simulink model "test_matlab_system_19"  (Simulink 10.0)
settings: Solver=FixedStepAuto  StartTime=0.0  StopTime=Config.simulationTime  FixedStep=Config.tStep  RelTol=1e-3
PostLoadFcn:
  | % Set path to the utility functions and to WBC library
  | import wbc.*
  | addpath(genpath('./src'));
  | addpath('./lib/RobotDynamicsWithContacts');
InitFcn:
  | init
undefined symbols (not defined in the file or in its folder): Config, confVisualizer
libraries: robotDynamicsWithContacts_lib x1
settings Model: Creator=giuseppe  LastModifiedBy=nunoguedelha
settings DataIOCC: SaveFormat=Dataset  ReturnWorkspaceOutputs=on
settings OptimizationCC: LifeSpan=auto
settings DebuggingCC: UnderspecifiedInitializationDetection=Simplified  MergeDetectMultiDrivingBlocksExec=error  SFUnexpectedBacktrackingDiag=error  SFNoUnconditionalDefaultTransitionDiag=error  SFExecutionAtInitializationDiag=warning  ArithmeticOperatorsInVariantConditions=error
settings HardwareCC: ProdBitPerPointer=64  ProdBitPerSizeT=64  ProdBitPerPtrDiffT=64  ProdLargestAtomicFloat=Float  ProdIntDivRoundTo=Zero  ProdEndianess=LittleEndian  ProdWordSize=64  ProdHWDeviceType=Intel->x86-64 (Windows64)
settings ModelReferenceCC: PropagateSignalLabelsOutOfModel=on
settings SFSimCC: SimUseLocalCustomCode=on  CustomCodeUndefinedFunction=FilterOut
settings RTWCC: RTWUseLocalCustomCode=on
settings CodeAppCC: StateflowObjectComments=off
settings GRTTargetCC: TargetLangStandard=C99 (ISO)  CombineOutputUpdateFcns=on  GRTInterface=off
settings ConfigComp: CovMetricSettings=dwe  CovHtmlReporting=off  CovSaveCumulativeToWorkspaceVar=off  CovSaveSingleToWorkspaceVar=off

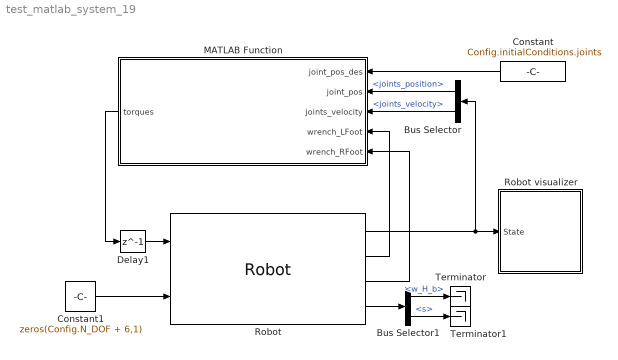
== system test_matlab_system_19 ==
  Bus Selector : BusSelector  OutputSignals=joints_position,joints_velocity
  Bus Selector1 : BusSelector  OutputSignals=w_H_b,s
  Constant : Constant  Value=Config.initialConditions.joints
  Constant1 : Constant  Value=zeros(Config.N_DOF + 6,1)
  Delay1 : Delay  DelayLength=1  InitialCondition=zeros(23,1)
  MATLAB Function : MATLAB Function  TreatAsAtomicUnit=on
  Robot : robotDynamicsWithContacts_lib/Robot  SystemSampleTime=-1  Latency=0  AutoFrameSizeCalculation=off
      settings: SourceProductName=RobotDynamicsWithContacts
  Robot visualizer : Subsystem  SystemSampleTime=confVisualizer.tStep
  Terminator : Terminator
  Terminator1 : Terminator
  wires:
  Constant1/1 -> Robot/2
  Bus Selector/1 -> MATLAB Function/2(joint_pos)  "<joints_position>"
  Bus Selector/2 -> MATLAB Function/3(joints_velocity)  "<joints_velocity>"
  Robot/1 -> Robot visualizer/1(State), Bus Selector/1
  Robot/2 -> MATLAB Function/4(wrench_LFoot)
  Robot/3 -> MATLAB Function/5(wrench_RFoot)
  Constant/1 -> MATLAB Function/1(joint_pos_des)
  MATLAB Function/1(torques) -> Delay1/1
  Delay1/1 -> Robot/1
  Robot/4 -> Bus Selector1/1
  Bus Selector1/2 -> Terminator1/1  "<s>"
  Bus Selector1/1 -> Terminator/1  "<w_H_b>"

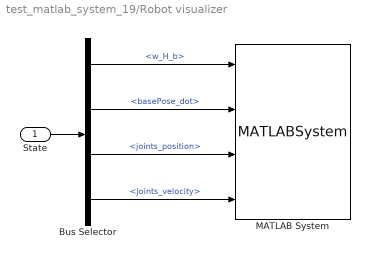
== system test_matlab_system_19/Robot visualizer ==
  State : Inport
  Bus Selector : BusSelector  OutputSignals=w_H_b,basePose_dot,joints_position,joints_velocity
  MATLAB System : MATLABSystem  System=Visualizer  config=confVisualizer  SimulateUsing=Interpreted execution
      mask Type: Visualizer
      mask Display:
      | disp(['Robot' char(10) 'Visualizer']);
      | port_label('input',1,'world_H_base');
      | port_label('input',2,'base_velocity');
      | port_label('input',3,'joints_positions');
      | port_label('input',4,'joints_velocity');
  wires:
  State/1 -> Bus Selector/1
  Bus Selector/1 -> MATLAB System/1  "<w_H_b>"
  Bus Selector/3 -> MATLAB System/3  "<joints_position>"
  Bus Selector/2 -> MATLAB System/2  "<basePose_dot>"
  Bus Selector/4 -> MATLAB System/4  "<joints_velocity>"

== matlab function MATLAB Function ==
  data: torques output double; joint_pos_des input double; joint_pos input double; joints_velocity input double; wrench_LFoot input double; wrench_RFoot input double
function torques = dummy_torque_control(joint_pos_des, joint_pos, joints_velocity, wrench_LFoot, wrench_RFoot)
    
    joints_pos_error = (joint_pos_des - joint_pos);
    
    KP = 0.1;
    KD = 2*sqrt(KP);
    
    torques = KP*(joints_pos_error) - KD*joints_velocity;
